simulink model "fm2"  (R2015a)
settings: Solver=ode45  StartTime=0.0  StopTime=0.03  MaxStep=1/60000  RelTol=1e-3
settings Model: Creator=baran_000  LastModifiedBy=baran_000

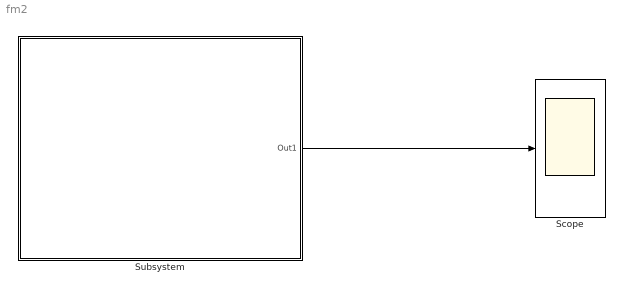
== system fm2 ==
  Scope : Scope
  Subsystem : Subsystem  mask(Fm Transmistter){fm=200, fc=1500}
      mask prompts: fm "Frequency of the Message"; fc "Frequency of the Carrier"
      mask help: This system generates the fm wave
      mask Help:
      | fm= frequency of Message
      | fc= Frequency of Carrier
      mask Display: image('b747.jpg')
  wires:
  Subsystem/1(Out1) -> Scope/1

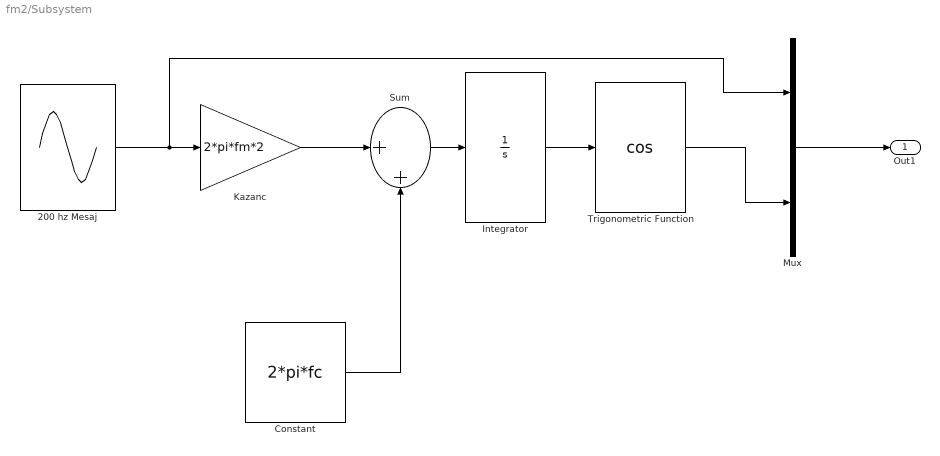
== system fm2/Subsystem ==
  "200 hz Mesaj " : Sin  Frequency=2*pi*fm  Phase=pi/2  SampleTime=0
  Constant : Constant  Value=2*pi*fc
  Integrator : Integrator
  Kazanc : Gain  Gain=2*pi*fm*2
  Mux : Mux  Inputs=2
  Sum : Sum  Inputs=|++
  Trigonometric Function : Trigonometry  Operator=cos
  Out1 : Outport
  wires:
  Trigonometric Function/1 -> Mux/2
  Kazanc/1 -> Sum/1
  Constant/1 -> Sum/2
  Sum/1 -> Integrator/1
  "200 hz Mesaj "/1 -> Mux/1, Kazanc/1
  Integrator/1 -> Trigonometric Function/1
  Mux/1 -> Out1/1
